simulink model "Problem1_4"  (R2018a)
settings: Solver=VariableStepAuto  StartTime=0  StopTime=30  RelTol=1e-3
settings Model: Creator=NIMA  LastModifiedBy=NIMA

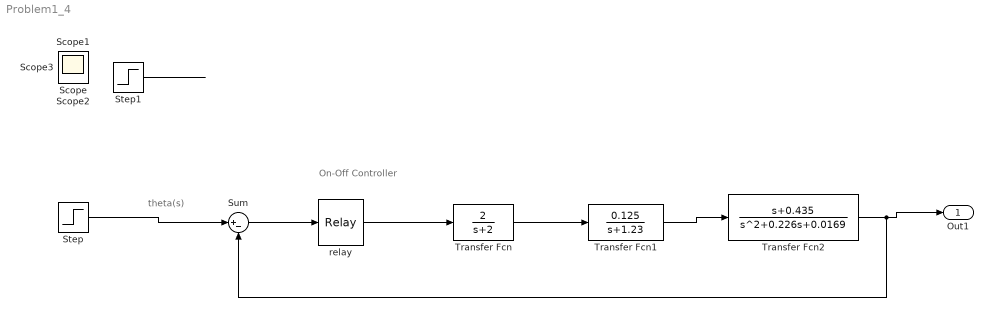
== system Problem1_4 ==
  note: On-Off
      | Controller
  note: theta(s)
  Step : Step  SampleTime=0
  Step1 : Step  Time=0  After=3  SampleTime=0
  Sum : Sum  Inputs=|+-
  Transfer Fcn : TransferFcn  Numerator=[2]  Denominator=[1 2]
  Transfer Fcn1 : TransferFcn  Numerator=[0.125]  Denominator=[1 1.23]
  Transfer Fcn2 : TransferFcn  Numerator=[1 0.435]  Denominator=[1 0.226 0.0169]
  relay : Relay  OnSwitchValue=0.001  OffSwitchValue=-0.001  OnOutputValue=1.15  OffOutputValue=-1.15
  Out1 : Outport
  Scope{,1..3} (4 alike) : Scope
  wires:
  Step/1 -> Sum/1
  Sum/1 -> relay/1
  relay/1 -> Transfer Fcn/1
  Transfer Fcn/1 -> Transfer Fcn1/1
  Transfer Fcn1/1 -> Transfer Fcn2/1
  Step1/1 -> ?
  Transfer Fcn2/1 -> Sum/2, Out1/1
